simulink subsystem "bh_COMPONENT_model_7dof_car_HAND"  (R2022b)
settings: Solver=VariableStepAuto  StartTime=0.0  StopTime=10.0  RelTol=1e-3
model mask{L_b=0, L_f=0, L_R=0, L_L=0, m_c=0, I_cZ=0, I_cX=0, m_bR=0, m_fR=0, m_bL=0, m_fL=0, k_bR=0, k_fR=0, k_bL=0, k_fL=0, k_bRG=0, k_fRG=0, k_bLG=0, k_fLG=0, c_bR=0, c_fR=0, c_bL=0, c_fL=0, c_bRG=0, c_fRG=0, c_bLG=0, c_fLG=0, IC_pos=zeros(7,1), IC_vel=zeros(7,1)}
  mask prompts: L_b "L_b   (m)"; L_f "L_f   (m)"; L_R "L_R   (m)"; L_L "L_L   (m)"; m_c "m_c     (kg)"; I_cZ "I_cZ      (kg.m^2)"; I_cX "I_cX      (kg.m2)"; m_bR "m_bR   (kg)"; m_fR "m_fR    (kg)"; m_bL "m_bL   (kg)"; m_fL "m_fL    (kg)"; k_bR "k_bR   (N/m)"; k_fR "k_fR   (N/m)"; k_bL "k_bL   (N/m)"; k_fL "k_fL    (N/m)"; k_bRG "k_bRG   (N/m)"; k_fRG "k_fRG   (N/m)"; k_bLG "k_bLG   (N/m)"; k_fLG "k_fLG    (N/m)"; c_bR "c_bR  (N.s/m)"; c_fR "c_fR  (N.s/m)"; c_bL "c_bL  (N.s/m)"; c_fL "c_fL  (N.s/m)"; c_bRG "c_bRG  (N.s/m)"; c_fRG "c_fRG  (N.s/m)"; c_bLG "c_bLG  (N.s/m)"; c_fLG "c_fLG  (N.s/m)"
settings Model: Creator=bhorton  LastModifiedBy=bhorton
settings DebuggingCC: UnconnectedInputMsg=warning  UnconnectedOutputMsg=warning  UnconnectedLineMsg=warning
settings ModelReferenceCC: EnableRefExpFcnMdlSchedulingChecks=on
settings RTWCC: DLArmComputeVersion=19.05

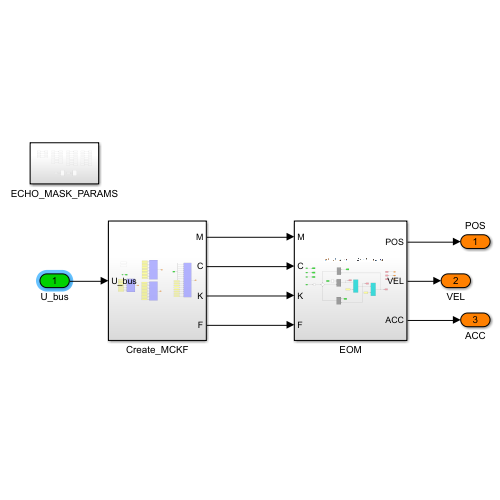
[thumbnail: Simulink's stored preview of the top-level diagram]
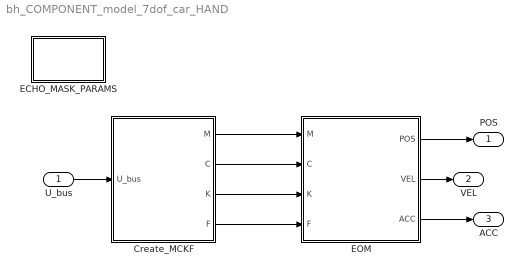
== system bh_COMPONENT_model_7dof_car_HAND ==
  U_bus : Inport
  Create_MCKF : Subsystem
  ECHO_MASK_PARAMS : Subsystem
  EOM : Subsystem
  POS : Outport
  VEL : Outport  Port=2
  ACC : Outport  Port=3
  wires:
  EOM/1(POS) -> POS/1
  EOM/2(VEL) -> VEL/1
  EOM/3(ACC) -> ACC/1
  U_bus/1 -> Create_MCKF/1(U_bus)
  Create_MCKF/1(M) -> EOM/1(M)
  Create_MCKF/2(C) -> EOM/2(C)
  Create_MCKF/3(K) -> EOM/3(K)
  Create_MCKF/4(F) -> EOM/4(F)

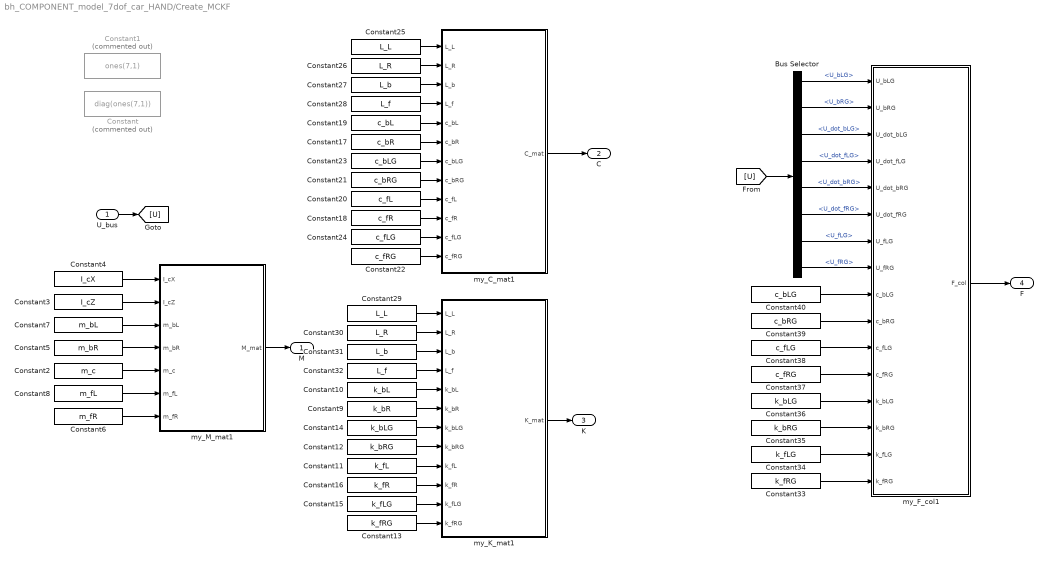
== system bh_COMPONENT_model_7dof_car_HAND/Create_MCKF ==
  U_bus : Inport
  Bus Selector : BusSelector  OutputSignals=U_bLG,U_bRG,U_dot_bLG,U_dot_fLG,U_dot_bRG,U_dot_fRG,U_fLG,U_fRG
  Constant : Constant  Commented=on  Value=diag(ones(7,1))  VectorParams1D=off
  Constant1 : Constant  Commented=on  Value=ones(7,1)  VectorParams1D=off
  Constant10 : Constant  Value=k_bL
  Constant11 : Constant  Value=k_fL
  Constant12 : Constant  Value=k_bRG
  Constant13 : Constant  Value=k_fRG
  Constant14 : Constant  Value=k_bLG
  Constant15 : Constant  Value=k_fLG
  Constant16 : Constant  Value=k_fR
  Constant17 : Constant  Value=c_bR
  Constant18 : Constant  Value=c_fR
  Constant19 : Constant  Value=c_bL
  Constant2 : Constant  Value=m_c
  Constant20 : Constant  Value=c_fL
  Constant21 : Constant  Value=c_bRG
  Constant22 : Constant  Value=c_fRG
  Constant23 : Constant  Value=c_bLG
  Constant24 : Constant  Value=c_fLG
  Constant25 : Constant  Value=L_L
  Constant26 : Constant  Value=L_R
  Constant27 : Constant  Value=L_b
  Constant28 : Constant  Value=L_f
  Constant29 : Constant  Value=L_L
  Constant3 : Constant  Value=I_cZ
  Constant30 : Constant  Value=L_R
  Constant31 : Constant  Value=L_b
  Constant32 : Constant  Value=L_f
  Constant33 : Constant  Value=k_fRG
  Constant34 : Constant  Value=k_fLG
  Constant35 : Constant  Value=k_bRG
  Constant36 : Constant  Value=k_bLG
  Constant37 : Constant  Value=c_fRG
  Constant38 : Constant  Value=c_fLG
  Constant39 : Constant  Value=c_bRG
  Constant4 : Constant  Value=I_cX
  Constant40 : Constant  Value=c_bLG
  Constant5 : Constant  Value=m_bR
  Constant6 : Constant  Value=m_fR
  Constant7 : Constant  Value=m_bL
  Constant8 : Constant  Value=m_fL
  Constant9 : Constant  Value=k_bR
  my_C_mat1 : MATLAB Function  TreatAsAtomicUnit=on
  my_F_col1 : MATLAB Function  TreatAsAtomicUnit=on
  my_K_mat1 : MATLAB Function  TreatAsAtomicUnit=on
  my_M_mat1 : MATLAB Function  TreatAsAtomicUnit=on
  M : Outport
  C : Outport  Port=2
  K : Outport  Port=3
  F : Outport  Port=4
  wires:
  my_F_col1/1(F_col) -> F/1
  my_K_mat1/1(K_mat) -> K/1
  my_C_mat1/1(C_mat) -> C/1
  my_M_mat1/1(M_mat) -> M/1
  Bus Selector/8 -> my_F_col1/8(U_fRG)  "<U_fRG>"
  Bus Selector/7 -> my_F_col1/7(U_fLG)  "<U_fLG>"
  Bus Selector/6 -> my_F_col1/6(U_dot_fRG)  "<U_dot_fRG>"
  Bus Selector/5 -> my_F_col1/5(U_dot_bRG)  "<U_dot_bRG>"
  Bus Selector/4 -> my_F_col1/4(U_dot_fLG)  "<U_dot_fLG>"
  Bus Selector/3 -> my_F_col1/3(U_dot_bLG)  "<U_dot_bLG>"
  Bus Selector/2 -> my_F_col1/2(U_bRG)  "<U_bRG>"
  Bus Selector/1 -> my_F_col1/1(U_bLG)  "<U_bLG>"
  [U] -> Bus Selector/1
  U_bus/1 -> [U]
  Constant40/1 -> my_F_col1/9(c_bLG)
  Constant39/1 -> my_F_col1/10(c_bRG)
  Constant38/1 -> my_F_col1/11(c_fLG)
  Constant37/1 -> my_F_col1/12(c_fRG)
  Constant36/1 -> my_F_col1/13(k_bLG)
  Constant35/1 -> my_F_col1/14(k_bRG)
  Constant33/1 -> my_F_col1/16(k_fRG)
  Constant34/1 -> my_F_col1/15(k_fLG)
  Constant13/1 -> my_K_mat1/12(k_fRG)
  Constant15/1 -> my_K_mat1/11(k_fLG)
  Constant16/1 -> my_K_mat1/10(k_fR)
  Constant11/1 -> my_K_mat1/9(k_fL)
  Constant12/1 -> my_K_mat1/8(k_bRG)
  Constant14/1 -> my_K_mat1/7(k_bLG)
  Constant9/1 -> my_K_mat1/6(k_bR)
  Constant10/1 -> my_K_mat1/5(k_bL)
  Constant32/1 -> my_K_mat1/4(L_f)
  Constant31/1 -> my_K_mat1/3(L_b)
  Constant30/1 -> my_K_mat1/2(L_R)
  Constant29/1 -> my_K_mat1/1(L_L)
  Constant22/1 -> my_C_mat1/12(c_fRG)
  Constant24/1 -> my_C_mat1/11(c_fLG)
  Constant18/1 -> my_C_mat1/10(c_fR)
  Constant20/1 -> my_C_mat1/9(c_fL)
  Constant21/1 -> my_C_mat1/8(c_bRG)
  Constant23/1 -> my_C_mat1/7(c_bLG)
  Constant17/1 -> my_C_mat1/6(c_bR)
  Constant19/1 -> my_C_mat1/5(c_bL)
  Constant28/1 -> my_C_mat1/4(L_f)
  Constant27/1 -> my_C_mat1/3(L_b)
  Constant26/1 -> my_C_mat1/2(L_R)
  Constant25/1 -> my_C_mat1/1(L_L)
  Constant3/1 -> my_M_mat1/2(I_cZ)
  Constant4/1 -> my_M_mat1/1(I_cX)
  Constant7/1 -> my_M_mat1/3(m_bL)
  Constant5/1 -> my_M_mat1/4(m_bR)
  Constant6/1 -> my_M_mat1/7(m_fR)
  Constant8/1 -> my_M_mat1/6(m_fL)
  Constant2/1 -> my_M_mat1/5(m_c)

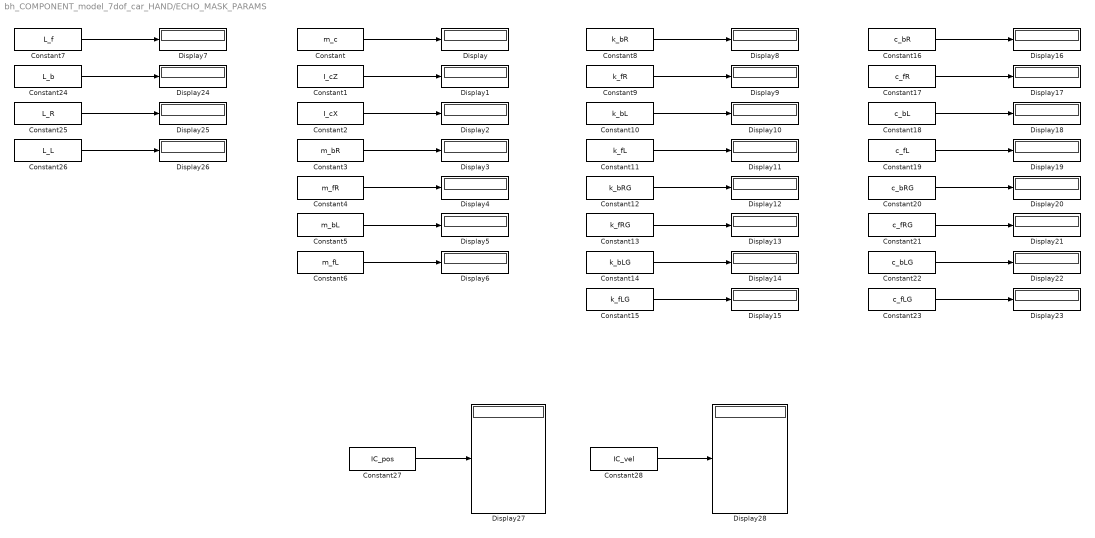
== system bh_COMPONENT_model_7dof_car_HAND/ECHO_MASK_PARAMS ==
  Constant : Constant  Value=m_c
  Constant1 : Constant  Value=I_cZ
  Constant10 : Constant  Value=k_bL
  Constant11 : Constant  Value=k_fL
  Constant12 : Constant  Value=k_bRG
  Constant13 : Constant  Value=k_fRG
  Constant14 : Constant  Value=k_bLG
  Constant15 : Constant  Value=k_fLG
  Constant16 : Constant  Value=c_bR
  Constant17 : Constant  Value=c_fR
  Constant18 : Constant  Value=c_bL
  Constant19 : Constant  Value=c_fL
  Constant2 : Constant  Value=I_cX
  Constant20 : Constant  Value=c_bRG
  Constant21 : Constant  Value=c_fRG
  Constant22 : Constant  Value=c_bLG
  Constant23 : Constant  Value=c_fLG
  Constant24 : Constant  Value=L_b
  Constant25 : Constant  Value=L_R
  Constant26 : Constant  Value=L_L
  Constant27 : Constant  Value=IC_pos
  Constant28 : Constant  Value=IC_vel
  Constant3 : Constant  Value=m_bR
  Constant4 : Constant  Value=m_fR
  Constant5 : Constant  Value=m_bL
  Constant6 : Constant  Value=m_fL
  Constant7 : Constant  Value=L_f
  Constant8 : Constant  Value=k_bR
  Constant9 : Constant  Value=k_fR
  Display{,1..28} (29 alike) : Display
  wires:
  Constant28/1 -> Display28/1
  Constant24/1 -> Display24/1
  Constant6/1 -> Display6/1
  Constant10/1 -> Display10/1
  Constant27/1 -> Display27/1
  Constant7/1 -> Display7/1
  Constant12/1 -> Display12/1
  Constant17/1 -> Display17/1
  Constant3/1 -> Display3/1
  Constant15/1 -> Display15/1
  Constant13/1 -> Display13/1
  Constant5/1 -> Display5/1
  Constant20/1 -> Display20/1
  Constant16/1 -> Display16/1
  Constant/1 -> Display/1
  Constant11/1 -> Display11/1
  Constant9/1 -> Display9/1
  Constant25/1 -> Display25/1
  Constant14/1 -> Display14/1
  Constant1/1 -> Display1/1
  Constant4/1 -> Display4/1
  Constant2/1 -> Display2/1
  Constant21/1 -> Display21/1
  Constant22/1 -> Display22/1
  Constant23/1 -> Display23/1
  Constant19/1 -> Display19/1
  Constant18/1 -> Display18/1
  Constant8/1 -> Display8/1
  Constant26/1 -> Display26/1

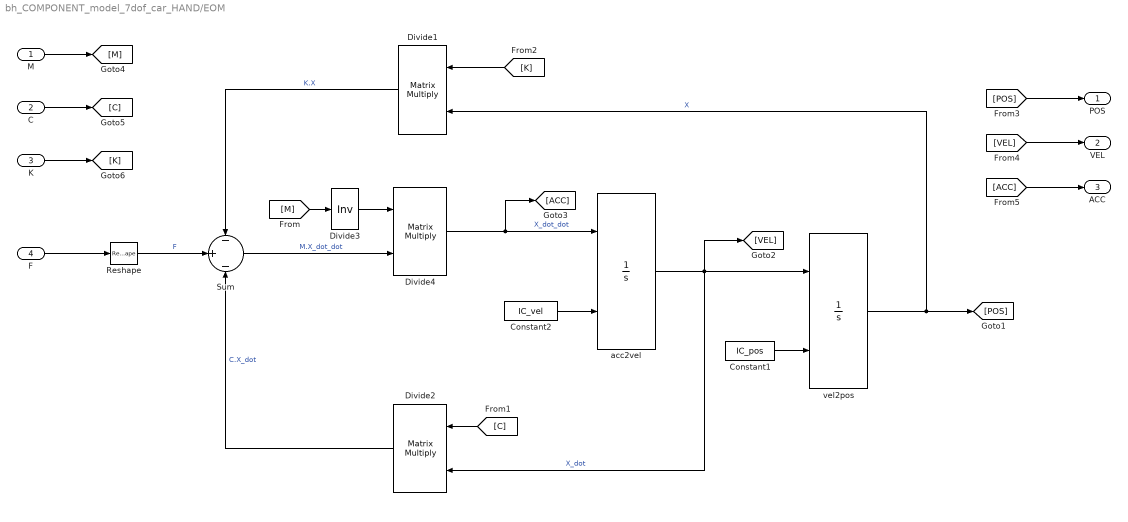
== system bh_COMPONENT_model_7dof_car_HAND/EOM ==
  M : Inport
  C : Inport  Port=2
  K : Inport  Port=3
  F : Inport  Port=4
  Constant1 : Constant  Value=IC_pos  VectorParams1D=off
  Constant2 : Constant  Value=IC_vel  VectorParams1D=off
  Divide1 : Product  Multiplication=Matrix(*)
  Divide2 : Product  Multiplication=Matrix(*)
  Divide3 : Product  Inputs=/  Multiplication=Matrix(*)
  Divide4 : Product  Multiplication=Matrix(*)
  Reshape : Reshape  OutputDimensionality=Column vector (2-D)
  Sum : Sum  Inputs=-|+|-
  acc2vel : Integrator  InitialConditionSource=external
  vel2pos : Integrator  InitialConditionSource=external
  POS : Outport
  VEL : Outport  Port=2
  ACC : Outport  Port=3
  wires:
  [POS] -> POS/1
  [VEL] -> VEL/1
  [ACC] -> ACC/1
  M/1 -> [M]
  C/1 -> [C]
  K/1 -> [K]
  Sum/1 -> Divide4/2  "M.X_dot_dot"
  Divide2/1 -> Sum/3  "C.X_dot"
  Reshape/1 -> Sum/2  "F"
  Divide1/1 -> Sum/1  "K.X"
  F/1 -> Reshape/1
  Divide4/1 -> [ACC], acc2vel/1  "X_dot_dot"
  vel2pos/1 -> [POS], Divide1/2  "X"
  Constant1/1 -> vel2pos/2
  Divide3/1 -> Divide4/1
  Constant2/1 -> acc2vel/2
  acc2vel/1 -> vel2pos/1, [VEL], Divide2/2  "X_dot"
  [K] -> Divide1/1
  [M] -> Divide3/1
  [C] -> Divide2/1

== matlab function bh_COMPONENT_model_7dof_car_HAND/Create_MCKF/my_K_mat1 ==
  data: L_L input; K_mat output; L_R input; L_b input; L_f input; k_bL input; k_bR input; k_bLG input; k_bRG input; k_fL input; k_fR input; k_fLG input; k_fRG input
function K_mat = my_K_mat(L_L,L_R,L_b,L_f,k_bL,k_bR,k_bLG,k_bRG,k_fL,k_fR,k_fLG,k_fRG)
%#codegen

%    This function was generated by the Symbolic Math Toolbox version 8.7.
%    02-Aug-2021 20:35:30

t2 = L_L.*k_bL;
t3 = L_L.*k_fL;
t4 = L_R.*k_bR;
t5 = L_R.*k_fR;
t6 = L_b.*k_bL;
t7 = L_b.*k_bR;
t8 = L_f.*k_fL;
t9 = L_f.*k_fR;
t10 = -k_bL;
t11 = -k_bR;
t12 = -k_fL;
t13 = -k_fR;
t14 = -t2;
t15 = -t3;
t16 = -t4;
t17 = -t5;
t18 = -t8;
t19 = -t9;
K_mat = reshape([k_bL+k_bR+k_fL+k_fR,-L_b.*(k_bL+k_bR)+L_f.*(k_fL+k_fR),L_L.*(k_bL+k_fL)-L_R.*(k_bR+k_fR),t11,t13,t10,t12,-t6-t7+t8+t9,L_b.*(t6+t7)+L_f.*(t8+t9),-L_L.*(t6+t18)+L_R.*(t7+t19),t7,t19,t6,t18,t2+t3+t16+t17,-L_b.*(t2+t16)+L_f.*(t3+t17),L_L.*(t2+t3)+L_R.*(t4+t5),t4,t5,t14,t15,t11,t7,t4,k_bR+k_bRG,0.0,0.0,0.0,t13,t19,t5,0.0,k_fR+k_fRG,0.0,0.0,t10,t6,t14,0.0,0.0,k_bL+k_bLG,0.0,t12,t18,t15,0.0,0.0,0.0,k_fL+k_fLG],[7,7]);

== matlab function bh_COMPONENT_model_7dof_car_HAND/Create_MCKF/my_C_mat1 ==
  data: L_L input; C_mat output; L_R input; L_b input; L_f input; c_bL input; c_bR input; c_bLG input; c_bRG input; c_fL input; c_fR input; c_fLG input; c_fRG input
function C_mat = my_C_mat(L_L,L_R,L_b,L_f,c_bL,c_bR,c_bLG,c_bRG,c_fL,c_fR,c_fLG,c_fRG)
%#codegen

%    This function was generated by the Symbolic Math Toolbox version 8.7.
%    02-Aug-2021 20:35:30

t2 = L_L.*c_bL;
t3 = L_L.*c_fL;
t4 = L_R.*c_bR;
t5 = L_R.*c_fR;
t6 = L_b.*c_bL;
t7 = L_b.*c_bR;
t8 = L_f.*c_fL;
t9 = L_f.*c_fR;
t10 = -c_bL;
t11 = -c_bR;
t12 = -c_fL;
t13 = -c_fR;
t14 = -t2;
t15 = -t3;
t16 = -t4;
t17 = -t5;
t18 = -t8;
t19 = -t9;
C_mat = reshape([c_bL+c_bR+c_fL+c_fR,-L_b.*(c_bL+c_bR)+L_f.*(c_fL+c_fR),L_L.*(c_bL+c_fL)-L_R.*(c_bR+c_fR),t11,t13,t10,t12,-t6-t7+t8+t9,L_b.*(t6+t7)+L_f.*(t8+t9),-L_L.*(t6+t18)+L_R.*(t7+t19),t7,t19,t6,t18,t2+t3+t16+t17,-L_b.*(t2+t16)+L_f.*(t3+t17),L_L.*(t2+t3)+L_R.*(t4+t5),t4,t5,t14,t15,t11,t7,t4,c_bR+c_bRG,0.0,0.0,0.0,t13,t19,t5,0.0,c_fR+c_fRG,0.0,0.0,t10,t6,t14,0.0,0.0,c_bL+c_bLG,0.0,t12,t18,t15,0.0,0.0,0.0,c_fL+c_fLG],[7,7]);

== matlab function bh_COMPONENT_model_7dof_car_HAND/Create_MCKF/my_F_col1 ==
  data: U_bLG input; F_col output; U_bRG input; U_dot_bLG input; U_dot_fLG input; U_dot_bRG input; U_dot_fRG input; U_fLG input; U_fRG input; c_bLG input; c_bRG input; c_fLG input; c_fRG input; k_bLG input; k_bRG input; k_fLG input; k_fRG input
function F_col = my_F_col(U_bLG,U_bRG,U_dot_bLG,U_dot_fLG,U_dot_bRG,U_dot_fRG,U_fLG,U_fRG,c_bLG,c_bRG,c_fLG,c_fRG,k_bLG,k_bRG,k_fLG,k_fRG)
%#codegen

%    This function was generated by the Symbolic Math Toolbox version 8.7.
%    02-Aug-2021 20:35:31

F_col = [0.0;0.0;0.0;U_dot_bRG.*c_bRG+U_bRG.*k_bRG;U_dot_fRG.*c_fRG+U_fRG.*k_fRG;U_dot_bLG.*c_bLG+U_bLG.*k_bLG;U_dot_fLG.*c_fLG+U_fLG.*k_fLG];

== matlab function bh_COMPONENT_model_7dof_car_HAND/Create_MCKF/my_M_mat1 ==
  data: I_cX input; M_mat output; I_cZ input; m_bL input; m_bR input; m_c input; m_fL input; m_fR input
function M_mat = my_M_mat(I_cX,I_cZ,m_bL,m_bR,m_c,m_fL,m_fR)
%#codegen

%    This function was generated by the Symbolic Math Toolbox version 8.7.
%    02-Aug-2021 20:35:29

M_mat = reshape([m_c,0.0,0.0,0.0,0.0,0.0,0.0,0.0,I_cZ,0.0,0.0,0.0,0.0,0.0,0.0,0.0,I_cX,0.0,0.0,0.0,0.0,0.0,0.0,0.0,m_bR,0.0,0.0,0.0,0.0,0.0,0.0,0.0,m_fR,0.0,0.0,0.0,0.0,0.0,0.0,0.0,m_bL,0.0,0.0,0.0,0.0,0.0,0.0,0.0,m_fL],[7,7]);
